simulink model "PDUSTM32"  (R2024b)
settings: Solver=FixedStepDiscrete  StartTime=0.0  StopTime=1  FixedStep=0.001  RelTol=1e-3  EnableMultiTasking=on
libraries: stm32blockslib x24, stm32f4xxblockslib x11, canmsglib x7, simulink x3, stm32h7xxblockslib x1
settings Model: STM32="{\"DigitalPortRead\":{\"ID\":\"PDUSTM32:620\"},\"SPIControllerTransfer\":[{\"ID\":\"PDUSTM32:616\"},{\"ID\":\"PDUSTM32:709\"},{\"ID\":\"PDUSTM32:716\"},{\"ID\":\"PDUSTM32:722\"},{\"ID\":\"PDUSTM32:728\"},{\"ID\":\"PDUSTM32:854\"},{\"ID\":\"PDUSTM32:855\"},{\"ID\":\"PDUSTM32:867\"},{\"ID\":\"PDUSTM32:868\"},{\"ID\":\"PDUSTM32:880\"},{\"ID\":\"PDUSTM32:881\"},{\"ID\":\"PDUSTM32:1012\"},{\"ID\":\"PDUSTM32:1013\"},{\"ID\":\"PDUSTM32:1014\"},{\"ID\":\"PDUSTM32:1015\"},{\"ID\":\"PDUSTM32:1016\"},{\"ID\":\"PDUSTM32:1017\"},{\"ID\":\"PDUSTM32:1018\"},{\"ID\":\"PDUSTM32:1019\"},{\"ID\":\"PDUSTM32:1077\"},{\"ID\":\"PDUSTM32:1078\"},{\"ID\":\"PDUSTM32:1090\"},{\"ID\":\"PDUSTM32:1109\"},{\"ID\":\"PDUSTM32:1110\"}],\"AnalogInputForH7\":{\"ID\":\"PDUSTM32:731\"},\"DigitalPortWrite\":[{\"ID\":\"PDUSTM32:809\"},{\"ID\":\"PDUSTM32:825\"},{\"ID\":\"PDUSTM32:826\"},{\"ID\":\"PDUSTM32:889\"},{\"ID\":\"PDUSTM32:921\"},{\"ID\":\"PDUSTM32:1091\"},{\"ID\":\"PDUSTM32:1092\"},{\"ID\":\"PDUSTM32:1093\"},{\"ID\":\"PDUSTM32:1094\"},{\"ID\":\"PDUSTM32:1095\"}]}"  Creator=will  LastModifiedBy=Will
settings SolverCC: AlgebraicLoopSolver=TrustRegion
settings DataIOCC: ReturnWorkspaceOutputs=off
settings OptimizationCC: DefaultParameterBehavior=Inlined  EnhancedBackFolding=on  PassReuseOutputArgsAs=Individual arguments  ZeroExternalMemoryAtStartup=off  ZeroInternalMemoryAtStartup=off  MaxStackSize=512  OptimizeBlockOrder=speed  DifferentSizesBufferReuse=on  OptimizationCustomize=off  EfficientTunableParamExpr=on
settings DebuggingCC: ParameterTunabilityLossMsg=error  UnconnectedInputMsg=warning  UnconnectedOutputMsg=warning  UnconnectedLineMsg=warning  ArithmeticOperatorsInVariantConditions=warning
settings HardwareCC: ProdBitPerPointer=32  ProdBitPerSizeT=32  ProdBitPerPtrDiffT=32  ProdLargestAtomicInteger=Long  ProdLargestAtomicFloat=Double  ProdWordSize=32  ProdLongLongMode=on  ProdHWDeviceType=ARM Compatible->ARM Cortex-M
settings ModelReferenceCC: EnableRefExpFcnMdlSchedulingChecks=on
settings SFSimCC: MATLABDynamicMemAlloc=off  CustomCodeUndefinedFunction=UseInterfaceOnly
settings RTWCC: Description=Embedded Coder  SystemTargetFile=ert.tlc  HardwareBoard=STM32H7xx Based (Single-core)  TemplateMakefile=ert_default_tmf  CustomHeaderCode="#include \"stm32h7xx_ll_tim.h\""  CustomInitializer=LL_TIM_EnableCounter(TIM2);  Toolchain=GNU Tools for ARM Embedded Processors  GPUComputeCapability=3.5
settings CodeAppCC: ForceParamTrailComments=on  IgnoreCustomStorageClasses=off  OperatorAnnotations=on  SimulinkDataObjDesc=on  SFDataObjDesc=on  InsertBlockDesc=on
settings ERTTargetCC: TargetLangStandard=C99 (ISO)  CodeReplacementLibrary=ARM Cortex-M  ExtModeTransport=3  ExtModeStaticAlloc=on  ExtModeStaticAllocSize=2048  ExtModeMexFile=ext_xcp  ExtModeIntrfLevel=Level2 - Open

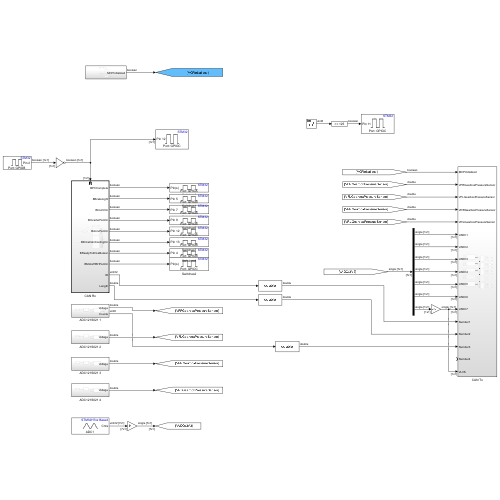
[thumbnail: Simulink's stored preview of the top-level diagram]
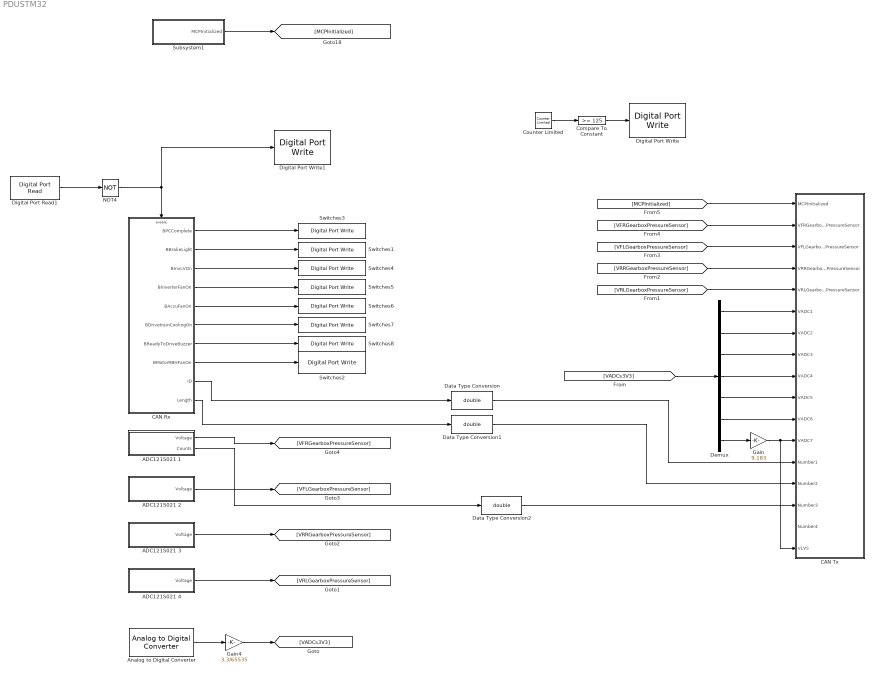
== system PDUSTM32 ==
  ADC121S021 1 : Subsystem
  ADC121S021 2 : Subsystem
  ADC121S021 3 : Subsystem
  ADC121S021 4 : Subsystem
  Analog to Digital Converter : stm32h7xxblockslib/Analog to Digital Converter  ADCModule=ADC1  ConversionGroup=Regular  TriggerMode=Read results only  NumberOfConversions=7  EnableBufferConv=off  BufferLength=1  OutputStatus=off  SampleTime=-1  EnableSimPort=off  hoistedMaskSrc=ECSoC/ECSimCodegen/Analog to Digital Converter
  CAN Rx : Subsystem  TreatAsAtomicUnit=on
  CAN Tx : Subsystem
  Compare To Constant : simulink/Logic and Bit Operations/Compare To Constant  relop=>=  const=125  OutDataTypeStr=boolean
  Counter Limited : simulink/Sources/Counter Limited  uplimit=250  tsamp=-1
  Data Type Conversion : DataTypeConversion  OutDataTypeStr=double  SaturateOnIntegerOverflow=off  RndMeth=Floor
  Data Type Conversion1 : DataTypeConversion  OutDataTypeStr=double  SaturateOnIntegerOverflow=off  RndMeth=Floor
  Data Type Conversion2 : DataTypeConversion  OutDataTypeStr=double  SaturateOnIntegerOverflow=off  RndMeth=Floor
  Demux : Demux  Outputs=7
  Digital Port Read1 : stm32f4xxblockslib/Digital Port Read  PortName=GPIOB  PinNumber=2  ReadOperation=on  IOAsArray=off  SampleTime=-1  EnableSimPort=off  hoistedMaskSrc=ECSoC/ECSimCodegen/Digital Port Read
      settings: LibrarySourceBlock=stm32f2xxblockslib/Digital Port Read
  Digital Port Write : stm32f4xxblockslib/Digital Port Write  PortName=GPIOC  PinNumber=11  ReadOperation=off  IOAsArray=off  EnableSimPort=off  hoistedMaskSrc=ECSoC/ECSimCodegen/Digital Port Write
      settings: LibrarySourceBlock=stm32h7xxblockslib/Digital Port Write
  Digital Port Write1 : stm32f4xxblockslib/Digital Port Write  PortName=GPIOC  PinNumber=12  ReadOperation=off  IOAsArray=off  EnableSimPort=off  hoistedMaskSrc=ECSoC/ECSimCodegen/Digital Port Write
      settings: LibrarySourceBlock=stm32h7xxblockslib/Digital Port Write
  Gain : Gain  Gain=9.183
  Gain4 : Gain  Gain=3.3/65535  OutDataTypeStr=single
  NOT4 : Logic  Operator=NOT  IconShape=distinctive  AllPortsSameDT=off  OutDataTypeStr=boolean
  Subsystem1 : Subsystem
  Switches1 : stm32f4xxblockslib/Digital Port Write  PortName=GPIOB  PinNumber=5  ReadOperation=off  IOAsArray=off  EnableSimPort=off  hoistedMaskSrc=ECSoC/ECSimCodegen/Digital Port Write
      settings: LibrarySourceBlock=stm32h7xxblockslib/Digital Port Write
  Switches2 : stm32f4xxblockslib/Digital Port Write  PortName=GPIOC  PinNumber=[2]  ReadOperation=off  IOAsArray=on  EnableSimPort=off  hoistedMaskSrc=ECSoC/ECSimCodegen/Digital Port Write
      settings: LibrarySourceBlock=stm32h7xxblockslib/Digital Port Write
  Switches3 : stm32f4xxblockslib/Digital Port Write  PortName=GPIOA  PinNumber=[12]  ReadOperation=off  IOAsArray=on  EnableSimPort=off  hoistedMaskSrc=ECSoC/ECSimCodegen/Digital Port Write
      settings: LibrarySourceBlock=stm32h7xxblockslib/Digital Port Write
  Switches4 : stm32f4xxblockslib/Digital Port Write  PortName=GPIOB  PinNumber=7  ReadOperation=off  IOAsArray=off  EnableSimPort=off  hoistedMaskSrc=ECSoC/ECSimCodegen/Digital Port Write
      settings: LibrarySourceBlock=stm32h7xxblockslib/Digital Port Write
  Switches5 : stm32f4xxblockslib/Digital Port Write  PortName=GPIOB  PinNumber=9  ReadOperation=off  IOAsArray=off  EnableSimPort=off  hoistedMaskSrc=ECSoC/ECSimCodegen/Digital Port Write
      settings: LibrarySourceBlock=stm32h7xxblockslib/Digital Port Write
  Switches6 : stm32f4xxblockslib/Digital Port Write  PortName=GPIOB  PinNumber=12  ReadOperation=off  IOAsArray=off  EnableSimPort=off  hoistedMaskSrc=ECSoC/ECSimCodegen/Digital Port Write
      settings: LibrarySourceBlock=stm32h7xxblockslib/Digital Port Write
  Switches7 : stm32f4xxblockslib/Digital Port Write  PortName=GPIOB  PinNumber=13  ReadOperation=off  IOAsArray=off  EnableSimPort=off  hoistedMaskSrc=ECSoC/ECSimCodegen/Digital Port Write
      settings: LibrarySourceBlock=stm32h7xxblockslib/Digital Port Write
  Switches8 : stm32f4xxblockslib/Digital Port Write  PortName=GPIOB  PinNumber=4  ReadOperation=off  IOAsArray=off  EnableSimPort=off  hoistedMaskSrc=ECSoC/ECSimCodegen/Digital Port Write
      settings: LibrarySourceBlock=stm32h7xxblockslib/Digital Port Write
  wires:
  NOT4/1 -> CAN Rx/Enable, Digital Port Write1/1
  Digital Port Read1/1 -> NOT4/1
  Analog to Digital Converter/1 -> Gain4/1
  Gain4/1 -> [VADCs3V3]
  [VADCs3V3] -> Demux/1
  ADC121S021 1/1(Voltage) -> [VFRGearboxPressureSensor]
  ADC121S021 2/1(Voltage) -> [VFLGearboxPressureSensor]
  ADC121S021 3/1(Voltage) -> [VRRGearboxPressureSensor]
  ADC121S021 4/1(Voltage) -> [VRLGearboxPressureSensor]
  [VFRGearboxPressureSensor] -> CAN Tx/2(VFRGearboxPressureSensor)
  [VFLGearboxPressureSensor] -> CAN Tx/3(VFLGearboxPressureSensor)
  [VRRGearboxPressureSensor] -> CAN Tx/4(VRRGearboxPressureSensor)
  CAN Rx/1(BPCComplete) -> Switches3/1
  [MCPInitialized] -> CAN Tx/1(MCPInitialized)
  CAN Rx/2(BBrakeLight) -> Switches1/1
  CAN Rx/8(BMotorRBHFanOn) -> Switches2/1
  Subsystem1/1(MCPInitialized) -> [MCPInitialized]
  Counter Limited/1 -> Compare To Constant/1
  Compare To Constant/1 -> Digital Port Write/1
  Demux/7 -> Gain/1
  Demux/6 -> CAN Tx/11(VADC6)
  Demux/5 -> CAN Tx/10(VADC5)
  Demux/4 -> CAN Tx/9(VADC4)
  Demux/3 -> CAN Tx/8(VADC3)
  Demux/2 -> CAN Tx/7(VADC2)
  Demux/1 -> CAN Tx/6(VADC1)
  Gain/1 -> CAN Tx/12(VADC7), CAN Tx/17(VLVS)
  CAN Rx/9(ID) -> Data Type Conversion/1
  [VRLGearboxPressureSensor] -> CAN Tx/5(VRLGearboxPressureSensor)
  Data Type Conversion/1 -> CAN Tx/13(Number1)
  CAN Rx/10(Length) -> Data Type Conversion1/1
  Data Type Conversion1/1 -> CAN Tx/14(Number2)
  CAN Rx/3(BInvLVOn) -> Switches4/1
  CAN Rx/4(BInverterFanOn) -> Switches5/1
  CAN Rx/5(BAccuFanOn) -> Switches6/1
  CAN Rx/6(BDrivetrainCoolingOn) -> Switches7/1
  CAN Rx/7(BReadyToDriveBuzzer) -> Switches8/1
  ADC121S021 1/2(Counts) -> Data Type Conversion2/1
  Data Type Conversion2/1 -> CAN Tx/15(Number3)

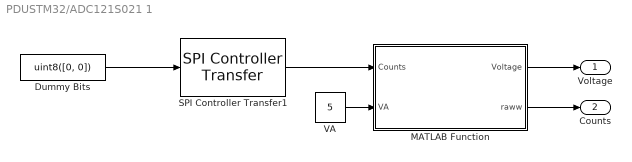
== system PDUSTM32/ADC121S021 1 ==
  Dummy Bits : Constant  Value=uint8([0, 0])
  MATLAB Function : MATLAB Function  TreatAsAtomicUnit=on
  SPI Controller Transfer1 : stm32blockslib/SPI Controller Transfer  Priority=2  SPIModuleSelect=SPI1  ClockPolarity=Low  ClockPhase=1 Edge  SPIModule=uint32(0)  Mode=Master  BusSpeed=uint32(1000000)  FirstBitToTransfer=Most significant bit (MSB)  ClockMode=0  BlockFunction=Transfer  EnableRegisterAddress=off  RegisterAddress=0  OutputDataType=uint8  OutputDataLength=1  OutputStatus=off  BlockingMode=on  Timeout=0.01  DataBits=8  UseCustomSSPin=Explicit GPIO calls  ActiveLowSSPin=Active low  Port_Select=GPIOA  Pin=0
      settings: LibrarySourceBlock=stm32h7xxblockslib/SPI Controller Transfer
  VA : Constant  Value=5  OutDataTypeStr=double
  Voltage : Outport  OutDataTypeStr=double
  Counts : Outport  Port=2  OutDataTypeStr=uint8
  wires:
  Dummy Bits/1 -> SPI Controller Transfer1/1
  SPI Controller Transfer1/1 -> MATLAB Function/1(Counts)
  VA/1 -> MATLAB Function/2(VA)
  MATLAB Function/1(Voltage) -> Voltage/1
  MATLAB Function/2(raww) -> Counts/1

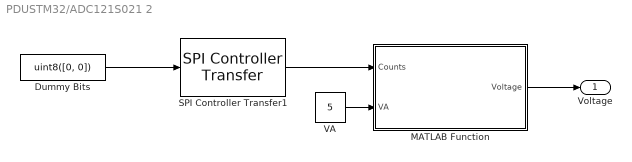
== system PDUSTM32/ADC121S021 2 ==
  Dummy Bits : Constant  Value=uint8([0, 0])
  MATLAB Function : MATLAB Function  TreatAsAtomicUnit=on
  SPI Controller Transfer1 : stm32blockslib/SPI Controller Transfer  Priority=2  SPIModuleSelect=SPI1  ClockPolarity=Low  ClockPhase=1 Edge  SPIModule=uint32(0)  Mode=Master  BusSpeed=uint32(1000000)  FirstBitToTransfer=Most significant bit (MSB)  ClockMode=0  BlockFunction=Transfer  EnableRegisterAddress=off  RegisterAddress=0  OutputDataType=uint8  OutputDataLength=1  OutputStatus=off  BlockingMode=on  Timeout=0.01  DataBits=8  UseCustomSSPin=Explicit GPIO calls  ActiveLowSSPin=Active low  Port_Select=GPIOA  Pin=1
      settings: LibrarySourceBlock=stm32h7xxblockslib/SPI Controller Transfer
  VA : Constant  Value=5
  Voltage : Outport  OutDataTypeStr=double
  wires:
  Dummy Bits/1 -> SPI Controller Transfer1/1
  SPI Controller Transfer1/1 -> MATLAB Function/1(Counts)
  VA/1 -> MATLAB Function/2(VA)
  MATLAB Function/1(Voltage) -> Voltage/1

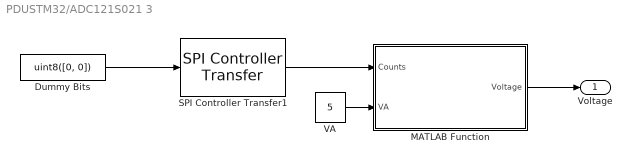
== system PDUSTM32/ADC121S021 3 ==
  Dummy Bits : Constant  Value=uint8([0, 0])
  MATLAB Function : MATLAB Function  TreatAsAtomicUnit=on
  SPI Controller Transfer1 : stm32blockslib/SPI Controller Transfer  Priority=2  SPIModuleSelect=SPI1  ClockPolarity=Low  ClockPhase=1 Edge  SPIModule=uint32(0)  Mode=Master  BusSpeed=uint32(1000000)  FirstBitToTransfer=Most significant bit (MSB)  ClockMode=0  BlockFunction=Transfer  EnableRegisterAddress=off  RegisterAddress=0  OutputDataType=uint8  OutputDataLength=1  OutputStatus=off  BlockingMode=on  Timeout=0.01  DataBits=8  UseCustomSSPin=Explicit GPIO calls  ActiveLowSSPin=Active low  Port_Select=GPIOA  Pin=2
      settings: LibrarySourceBlock=stm32h7xxblockslib/SPI Controller Transfer
  VA : Constant  Value=5
  Voltage : Outport  OutDataTypeStr=double
  wires:
  Dummy Bits/1 -> SPI Controller Transfer1/1
  SPI Controller Transfer1/1 -> MATLAB Function/1(Counts)
  VA/1 -> MATLAB Function/2(VA)
  MATLAB Function/1(Voltage) -> Voltage/1

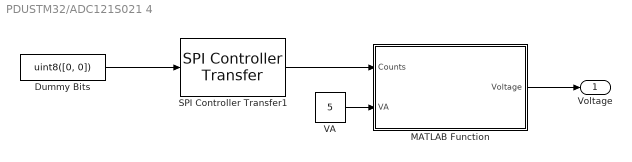
== system PDUSTM32/ADC121S021 4 ==
  Dummy Bits : Constant  Value=uint8([0, 0])
  MATLAB Function : MATLAB Function  TreatAsAtomicUnit=on
  SPI Controller Transfer1 : stm32blockslib/SPI Controller Transfer  Priority=2  SPIModuleSelect=SPI1  ClockPolarity=Low  ClockPhase=1 Edge  SPIModule=uint32(0)  Mode=Master  BusSpeed=uint32(1000000)  FirstBitToTransfer=Most significant bit (MSB)  ClockMode=0  BlockFunction=Transfer  EnableRegisterAddress=off  RegisterAddress=0  OutputDataType=uint8  OutputDataLength=1  OutputStatus=off  BlockingMode=on  Timeout=0.01  DataBits=8  UseCustomSSPin=Explicit GPIO calls  ActiveLowSSPin=Active low  Port_Select=GPIOB  Pin=10
      settings: LibrarySourceBlock=stm32h7xxblockslib/SPI Controller Transfer
  VA : Constant  Value=5
  Voltage : Outport  OutDataTypeStr=double
  wires:
  Dummy Bits/1 -> SPI Controller Transfer1/1
  SPI Controller Transfer1/1 -> MATLAB Function/1(Counts)
  VA/1 -> MATLAB Function/2(VA)
  MATLAB Function/1(Voltage) -> Voltage/1

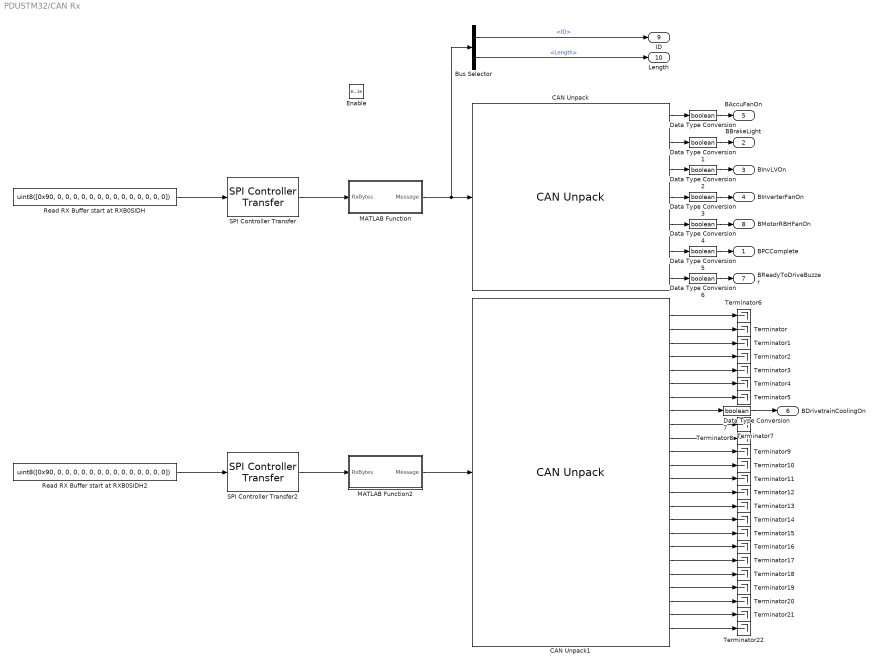
== system PDUSTM32/CAN Rx ==
  Enable : EnablePort
  Bus Selector : BusSelector  OutputSignals=ID,Length
  CAN Unpack : canmsglib/CAN Unpack  CANdbFile=C:\Users\oxbro\Documents\STM32CustomProjects\PDUSTM32\CAN3_28.06.26.dbc  MsgList=VCU_PDMReq  MsgName=VCU_PDMReq  MsgIDType=Standard (11-bit identifier)  MsgIdentifier=1539  MsgLength=7  SignalInfo={'BAccuFanOn','24','1','LE','unsigned','Standard','0','1','0','0','1';'BBrakeLight','0','1','LE','unsigned','Standard','0','1','0','0','1';'BInvLVOn','32','1','LE','unsigned','Standard','0','1','0','0','1';'BInverterFanOn','8','1','LE','unsigned','Standard','0','1','0','0','1';'BMotorRBHFanOn','16','1','LE','unsigned','Standard','0','1','0','0','1';'BPCComplete','40','1','LE','unsigned','Standard','0','1','0','0','1';'BReadyToDriveBuzzer','48','1','LE','unsigned','Standard','0','1','0','0','1'}  IDPort=off  TimestampPort=off  ErrorPort=off  RemotePort=off  LengthPort=off  StatusPort=off  ApplyMinMax=off
      settings: LibrarySourceBlock=stmutilitieslib/CAN Unpack  DataFormat=CANdb specified signals
  CAN Unpack1 : canmsglib/CAN Unpack  CANdbFile=C:\Users\will\Desktop\STM32Projects\PDUSTM32\CAN3_28.06.26.dbc  MsgList=VCU_1s_Frame4  MsgName=VCU_1s_Frame4  MsgIDType=Standard (11-bit identifier)  MsgIdentifier=419  MsgLength=6  SignalInfo={'BBMSP0A0COut','32','1','LE','unsigned','Standard','0','1','0','0','1';'BBMSP0A0EOut','33','1','LE','unsigned','Standard','0','1','0','0','1';'BBMSP0A10Out','34','1','LE','unsigned','Standard','0','1','0','0','1';'BBMSP0A80Out','35','1','LE','unsigned','Standard','0','1','0','0','1';'BBMSP0AC0Out','36','1','LE','unsigned','Standard','0','1','0','0','1';'BBMSP0AFAOut','37','1','LE','unsigned','Standard','0','1','0','0','1';'BBalancingOnOut','31','1','LE','unsigned','Standard','0','1','0','0','1';'BDrivetrainCoolingOn','1','1','LE','unsigned','Standard','0','1','0','0','1';'BDrivetrainCoolingOnEM','5','1','LE','unsigned','Standard','0','1','0','0','1';'BDrivetrainCoolingOnOW','6','2','LE','unsigned','Standard','0','1','-1','-1','2';'BEMSOn','13','1','LE','unsigned','Standard','0','1','0','0','1';'BEMSOnEM','14','1','LE','unsigned','Standard','0','1','0','0','1';'BEMSOnOW','15','2','LE','unsigned','Standard','0','1','-1','-1','2';'BSpinningModeOn','17','1','LE','unsigned','Standard','0','1','0','0','1';'BSpinningModeOnEM','18','1','LE','unsigned','Standard','0','1','0','0','1';'BSpinningModeOnOW','19','2','LE','unsigned','Standard','0','1','-1','-1','2';'BTCOn','9','1','LE','unsigned','Standard','0','1','0','0','1';'BTCOnEM','10','1','LE','unsigned','Standard','0','1','0','0','1';'BTCOnOW','11','2','LE','unsigned','Standard','0','1','-1','-1','2';'BTVOnEM','0','1','LE','unsigned','Standard','0','1','0','0','1';'BTVOnOW','2','2','LE','unsigned','Standard','0','1','-1','-1','2';'NEventMode','44','4','LE','unsigned','Standard','0','1','0','0','15';'NLap','38','6','LE','unsigned','Standard','0','1','0','0','63';'rSoE','21','10','LE','unsigned','Standard','0','0.1','0','0','102.3'}  IDPort=off  TimestampPort=off  ErrorPort=off  RemotePort=off  LengthPort=off  StatusPort=off  ApplyMinMax=off
      settings: LibrarySourceBlock=stmutilitieslib/CAN Unpack  DataFormat=CANdb specified signals
  Data Type Conversion{,1..7} (8 alike) : DataTypeConversion  OutDataTypeStr=boolean  SaturateOnIntegerOverflow=off  RndMeth=Floor
  MATLAB Function : MATLAB Function  TreatAsAtomicUnit=on
  MATLAB Function2 : MATLAB Function  TreatAsAtomicUnit=on
  Read RX Buffer start at RXB0SIDH : Constant  Value=uint8([0x90, 0, 0, 0, 0, 0, 0, 0, 0, 0, 0, 0, 0, 0, 0])
  Read RX Buffer start at RXB0SIDH2 : Constant  Value=uint8([0x90, 0, 0, 0, 0, 0, 0, 0, 0, 0, 0, 0, 0, 0, 0])
  SPI Controller Transfer : stm32blockslib/SPI Controller Transfer  Priority=1  SPIModuleSelect=SPI1  ClockPolarity=Low  ClockPhase=1 Edge  SPIModule=uint32(0)  Mode=Master  BusSpeed=uint32(1000000)  FirstBitToTransfer=Most significant bit (MSB)  ClockMode=0  BlockFunction=Transfer  EnableRegisterAddress=off  RegisterAddress=0  OutputDataType=uint8  OutputDataLength=1  OutputStatus=off  BlockingMode=on  Timeout=0.01  DataBits=8  UseCustomSSPin=Explicit GPIO calls  ActiveLowSSPin=Active low  Port_Select=GPIOB  Pin=14
      settings: LibrarySourceBlock=stm32h7xxblockslib/SPI Controller Transfer
  SPI Controller Transfer2 : stm32blockslib/SPI Controller Transfer  Priority=1  SPIModuleSelect=SPI1  ClockPolarity=Low  ClockPhase=1 Edge  SPIModule=uint32(0)  Mode=Master  BusSpeed=uint32(1000000)  FirstBitToTransfer=Most significant bit (MSB)  ClockMode=0  BlockFunction=Transfer  EnableRegisterAddress=off  RegisterAddress=0  OutputDataType=uint8  OutputDataLength=1  OutputStatus=off  BlockingMode=on  Timeout=0.01  DataBits=8  UseCustomSSPin=Explicit GPIO calls  ActiveLowSSPin=Active low  Port_Select=GPIOB  Pin=14
      settings: LibrarySourceBlock=stm32h7xxblockslib/SPI Controller Transfer
  Terminator{,1..22} (23 alike) : Terminator
  BPCComplete : Outport  OutDataTypeStr=boolean
  BBrakeLight : Outport  Port=2  OutDataTypeStr=boolean
  BInvLVOn : Outport  Port=3  OutDataTypeStr=boolean
  BInverterFanOn : Outport  Port=4  OutDataTypeStr=boolean
  BAccuFanOn : Outport  Port=5  OutDataTypeStr=boolean
  BDrivetrainCoolingOn : Outport  Port=6  OutDataTypeStr=boolean
  BReadyToDriveBuzzer : Outport  Port=7  OutDataTypeStr=boolean
  BMotorRBHFanOn : Outport  Port=8  OutDataTypeStr=boolean
  ID : Outport  Port=9
  Length : Outport  Port=10
  wires:
  Read RX Buffer start at RXB0SIDH/1 -> SPI Controller Transfer/1
  SPI Controller Transfer/1 -> MATLAB Function/1(RxBytes)
  MATLAB Function/1(Message) -> Bus Selector/1, CAN Unpack/1
  CAN Unpack/1 -> Data Type Conversion/1
  CAN Unpack/2 -> Data Type Conversion1/1
  CAN Unpack1/2 -> Terminator/1
  CAN Unpack1/3 -> Terminator1/1
  CAN Unpack1/4 -> Terminator2/1
  CAN Unpack1/5 -> Terminator3/1
  CAN Unpack1/6 -> Terminator4/1
  CAN Unpack1/7 -> Terminator5/1
  CAN Unpack1/9 -> Terminator7/1
  CAN Unpack1/10 -> Terminator8/1
  CAN Unpack1/19 -> Terminator17/1
  CAN Unpack1/18 -> Terminator16/1
  CAN Unpack1/17 -> Terminator15/1
  CAN Unpack1/16 -> Terminator14/1
  CAN Unpack1/15 -> Terminator13/1
  CAN Unpack1/14 -> Terminator12/1
  CAN Unpack1/13 -> Terminator11/1
  CAN Unpack1/12 -> Terminator10/1
  CAN Unpack1/20 -> Terminator18/1
  CAN Unpack1/21 -> Terminator19/1
  CAN Unpack1/22 -> Terminator20/1
  CAN Unpack1/23 -> Terminator21/1
  CAN Unpack1/24 -> Terminator22/1
  CAN Unpack1/11 -> Terminator9/1
  CAN Unpack1/1 -> Terminator6/1
  Data Type Conversion/1 -> BAccuFanOn/1
  Data Type Conversion1/1 -> BBrakeLight/1
  Data Type Conversion2/1 -> BInvLVOn/1
  Data Type Conversion3/1 -> BInverterFanOn/1
  Data Type Conversion4/1 -> BMotorRBHFanOn/1
  Data Type Conversion6/1 -> BReadyToDriveBuzzer/1
  Data Type Conversion7/1 -> BDrivetrainCoolingOn/1
  Data Type Conversion5/1 -> BPCComplete/1
  CAN Unpack1/8 -> Data Type Conversion7/1
  CAN Unpack/7 -> Data Type Conversion6/1
  Bus Selector/1 -> ID/1  "<ID>"
  Bus Selector/2 -> Length/1  "<Length>"
  Read RX Buffer start at RXB0SIDH2/1 -> SPI Controller Transfer2/1
  SPI Controller Transfer2/1 -> MATLAB Function2/1(RxBytes)
  MATLAB Function2/1(Message) -> CAN Unpack1/1
  CAN Unpack/3 -> Data Type Conversion2/1
  CAN Unpack/4 -> Data Type Conversion3/1
  CAN Unpack/5 -> Data Type Conversion4/1
  CAN Unpack/6 -> Data Type Conversion5/1

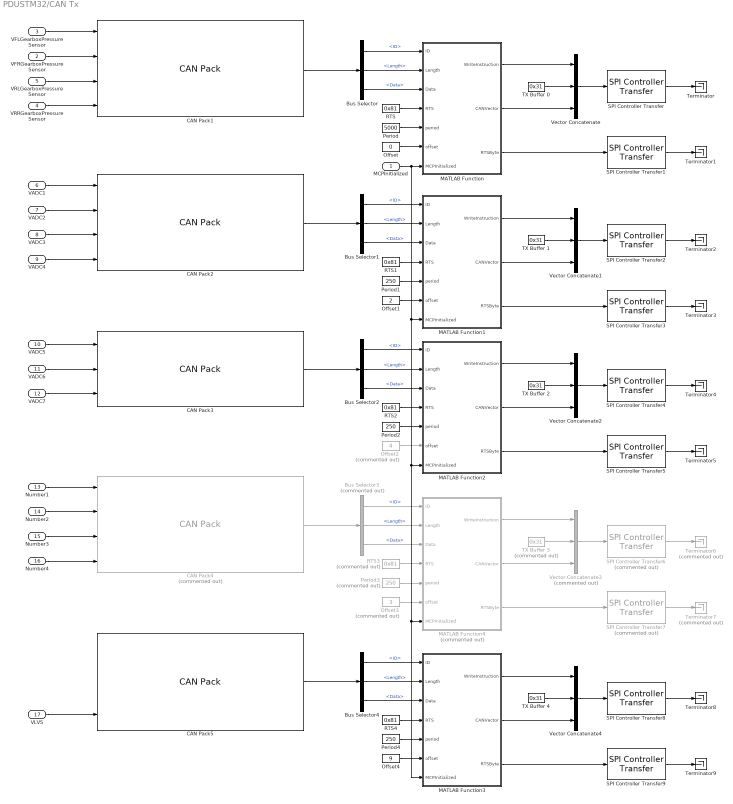
== system PDUSTM32/CAN Tx ==
  MCPInitialized : Inport
  VFRGearboxPressureSensor : Inport  Port=2
  VFLGearboxPressureSensor : Inport  Port=3
  VRRGearboxPressureSensor : Inport  Port=4
  VRLGearboxPressureSensor : Inport  Port=5
  VADC1 : Inport  Port=6
  VADC2 : Inport  Port=7
  VADC3 : Inport  Port=8
  VADC4 : Inport  Port=9
  VADC5 : Inport  Port=10
  VADC6 : Inport  Port=11
  VADC7 : Inport  Port=12
  Number1 : Inport  Port=13
  Number2 : Inport  Port=14
  Number3 : Inport  Port=15
  Number4 : Inport  Port=16
  VLVS : Inport  Port=17
  Bus Selector{,1..2,4} (4 alike) : BusSelector  OutputSignals=ID,Length,Data
  Bus Selector3 : BusSelector  Commented=on  OutputSignals=ID,Length,Data
  CAN Pack1 : canmsglib/CAN Pack  CANdbFile=C:\Users\oxbro\Documents\STM32CustomProjects\PDUSTM32\ADCTest.dbc  MsgList=GearboxPressures  MsgName=GearboxPressures  MsgIDType=Standard (11-bit identifier)  MsgIdentifier=105  CANIDInput=off  MsgLength=8  Remote=off  ApplyMinMax=off  BusOutput=on  SignalInfo={'VFLGearboxPressureSensor','0','12','LE','unsigned','Standard','0','0.0012211','0','0','5.0004';'VFRGearboxPressureSensor','16','12','LE','unsigned','Standard','0','0.0012211','0','0','5.0004';'VRLGearboxPressureSensor','32','12','LE','unsigned','Standard','0','0.0012211','0','0','5.0004';'VRRGearboxPressureSensor','48','12','LE','unsigned','Standard','0','0.0012211','0','0','5.0004'}
      settings: LibrarySourceBlock=stmutilitieslib/CAN Pack  DataFormat=CANdb specified signals
  CAN Pack2 : canmsglib/CAN Pack  CANdbFile=C:\Users\oxbro\Documents\STM32CustomProjects\PDUSTM32\ADCTest.dbc  MsgList=ADCs1  MsgName=ADCs1  MsgIDType=Standard (11-bit identifier)  MsgIdentifier=5  CANIDInput=off  MsgLength=8  Remote=off  ApplyMinMax=off  BusOutput=on  SignalInfo={'VADC1','0','16','LE','unsigned','Standard','0','5.04e-05','0','0','3.303';'VADC2','16','16','LE','unsigned','Standard','0','5.04e-05','0','0','3.303';'VADC3','32','16','LE','unsigned','Standard','0','5.04e-05','0','0','3.303';'VADC4','48','16','LE','unsigned','Standard','0','5.04e-05','0','0','3.303'}
      settings: LibrarySourceBlock=stmutilitieslib/CAN Pack  DataFormat=CANdb specified signals
  CAN Pack3 : canmsglib/CAN Pack  CANdbFile=C:\Users\oxbro\Documents\STM32CustomProjects\PDUSTM32\ADCTest.dbc  MsgList=ADCs2  MsgName=ADCs2  MsgIDType=Standard (11-bit identifier)  MsgIdentifier=66  CANIDInput=off  MsgLength=6  Remote=off  ApplyMinMax=off  BusOutput=on  SignalInfo={'VADC5','0','16','LE','unsigned','Standard','0','5.04e-05','0','0','3.303';'VADC6','16','16','LE','unsigned','Standard','0','5.04e-05','0','0','3.303';'VLVSystem','32','16','LE','unsigned','Standard','0','0.00046327','0','0','30.3604'}
      settings: LibrarySourceBlock=stmutilitieslib/CAN Pack  DataFormat=CANdb specified signals
  CAN Pack4 : canmsglib/CAN Pack  Commented=on  CANdbFile=C:\Users\oxbro\Documents\STM32CustomProjects\PDUSTM32\ADCTest.dbc  MsgList=Numbers  MsgName=Numbers  MsgIDType=Standard (11-bit identifier)  MsgIdentifier=0  CANIDInput=off  MsgLength=8  Remote=off  ApplyMinMax=off  BusOutput=on  SignalInfo={'Number1','0','16','LE','signed','Standard','0','1','0','-32768','32767';'Number2','16','16','LE','signed','Standard','0','1','0','-32768','32767';'Number3','32','16','LE','signed','Standard','0','1','0','-32768','32767';'Number4','48','16','LE','signed','Standard','0','1','0','-32768','32767'}
      settings: LibrarySourceBlock=stmutilitieslib/CAN Pack  DataFormat=CANdb specified signals
  CAN Pack5 : canmsglib/CAN Pack  CANdbFile=C:\Users\Will\Desktop\OBR\Embedded\PDUSTM32\CAN3_28.06.26.dbc  MsgList=PDM_Data  MsgName=PDM_Data  MsgIDType=Standard (11-bit identifier)  MsgIdentifier=1328  CANIDInput=off  MsgLength=8  Remote=off  ApplyMinMax=off  BusOutput=on  SignalInfo={'ILVS','8','8','LE','unsigned','Standard','0','1','0','0','255';'TPDM','16','8','LE','unsigned','Standard','0','1','0','0','255';'VLVS','0','8','LE','unsigned','Standard','0','0.1216','0','0','31.008'}
      settings: LibrarySourceBlock=stmutilitieslib/CAN Pack  DataFormat=CANdb specified signals
  MATLAB Function : MATLAB Function  TreatAsAtomicUnit=on
  MATLAB Function1 : MATLAB Function  TreatAsAtomicUnit=on
  MATLAB Function2 : MATLAB Function  TreatAsAtomicUnit=on
  MATLAB Function3 : MATLAB Function  TreatAsAtomicUnit=on
  MATLAB Function4 : MATLAB Function  Commented=on  TreatAsAtomicUnit=on
  Offset : Constant  Value=0  OutDataTypeStr=uint16  SampleTime=-1
  Offset1 : Constant  Value=2  OutDataTypeStr=uint16  SampleTime=-1
  Offset2 : Constant  Commented=on  Value=4  OutDataTypeStr=uint16  SampleTime=-1
  Offset3 : Constant  Commented=on  Value=3  OutDataTypeStr=uint16  SampleTime=-1
  Offset4 : Constant  Value=9  OutDataTypeStr=uint16  SampleTime=-1
  Period : Constant  Value=5000  OutDataTypeStr=uint16  SampleTime=-1
  Period1 : Constant  Value=250  OutDataTypeStr=uint16  SampleTime=-1
  Period2 : Constant  Value=250  OutDataTypeStr=uint16  SampleTime=-1
  Period3 : Constant  Commented=on  Value=250  OutDataTypeStr=uint16  SampleTime=-1
  Period4 : Constant  Value=250  OutDataTypeStr=uint16  SampleTime=-1
  RTS{,1..2,4} (4 alike) : Constant  Value=0x81  OutDataTypeStr=uint8  SampleTime=-1
  RTS3 : Constant  Commented=on  Value=0x81  OutDataTypeStr=uint8  SampleTime=-1
  SPI Controller Transfer{,2,4,8} (4 alike) : stm32blockslib/SPI Controller Transfer  Priority=1  SPIModuleSelect=SPI1  ClockPolarity=Low  ClockPhase=1 Edge  SPIModule=uint32(0)  Mode=Master  BusSpeed=uint32(1000000)  FirstBitToTransfer=Most significant bit (MSB)  ClockMode=0  BlockFunction=Transfer  EnableRegisterAddress=off  RegisterAddress=0  OutputDataType=uint8  OutputDataLength=1  OutputStatus=off  BlockingMode=off  Timeout=0.01  DataBits=8  UseCustomSSPin=Explicit GPIO calls  ActiveLowSSPin=Active low  Port_Select=GPIOB  Pin=14
      settings: LibrarySourceBlock=stm32h7xxblockslib/SPI Controller Transfer
  SPI Controller Transfer{1,3,5,9} (4 alike) : stm32blockslib/SPI Controller Transfer  Priority=2  SPIModuleSelect=SPI1  ClockPolarity=Low  ClockPhase=1 Edge  SPIModule=uint32(0)  Mode=Master  BusSpeed=uint32(1000000)  FirstBitToTransfer=Most significant bit (MSB)  ClockMode=0  BlockFunction=Transfer  EnableRegisterAddress=off  RegisterAddress=0  OutputDataType=uint8  OutputDataLength=1  OutputStatus=off  BlockingMode=off  Timeout=0.01  DataBits=8  UseCustomSSPin=Explicit GPIO calls  ActiveLowSSPin=Active low  Port_Select=GPIOB  Pin=14
      settings: LibrarySourceBlock=stm32h7xxblockslib/SPI Controller Transfer
  SPI Controller Transfer6 : stm32blockslib/SPI Controller Transfer  Priority=1  Commented=on  SPIModuleSelect=SPI1  ClockPolarity=Low  ClockPhase=1 Edge  SPIModule=uint32(0)  Mode=Master  BusSpeed=uint32(1000000)  FirstBitToTransfer=Most significant bit (MSB)  ClockMode=0  BlockFunction=Transfer  EnableRegisterAddress=off  RegisterAddress=0  OutputDataType=uint8  OutputDataLength=1  OutputStatus=off  BlockingMode=off  Timeout=0.01  DataBits=8  UseCustomSSPin=Explicit GPIO calls  ActiveLowSSPin=Active low  Port_Select=GPIOB  Pin=14
      settings: LibrarySourceBlock=stm32h7xxblockslib/SPI Controller Transfer
  SPI Controller Transfer7 : stm32blockslib/SPI Controller Transfer  Priority=2  Commented=on  SPIModuleSelect=SPI1  ClockPolarity=Low  ClockPhase=1 Edge  SPIModule=uint32(0)  Mode=Master  BusSpeed=uint32(1000000)  FirstBitToTransfer=Most significant bit (MSB)  ClockMode=0  BlockFunction=Transfer  EnableRegisterAddress=off  RegisterAddress=0  OutputDataType=uint8  OutputDataLength=1  OutputStatus=off  BlockingMode=off  Timeout=0.01  DataBits=8  UseCustomSSPin=Explicit GPIO calls  ActiveLowSSPin=Active low  Port_Select=GPIOB  Pin=14
      settings: LibrarySourceBlock=stm32h7xxblockslib/SPI Controller Transfer
  TX Buffer {0..2,4} (4 alike) : Constant  Value=0x31  OutDataTypeStr=uint8  SampleTime=-1
  TX Buffer 3 : Constant  Commented=on  Value=0x31  OutDataTypeStr=uint8  SampleTime=-1
  Terminator{,1..5,8..9} (8 alike) : Terminator
  Terminator6 : Terminator  Commented=on
  Terminator7 : Terminator  Commented=on
  Vector Concatenate{,1..2,4} (4 alike) : Concatenate  NumInputs=3
  Vector Concatenate3 : Concatenate  Commented=on  NumInputs=3
  wires:
  SPI Controller Transfer/1 -> Terminator/1
  MATLAB Function/1(WriteInstruction) -> Vector Concatenate/1
  RTS/1 -> MATLAB Function/4(RTS)
  MATLAB Function/2(CANVector) -> Vector Concatenate/3
  SPI Controller Transfer1/1 -> Terminator1/1
  Bus Selector/1 -> MATLAB Function/1(ID)  "<ID>"
  Vector Concatenate/1 -> SPI Controller Transfer/1
  TX Buffer 0/1 -> Vector Concatenate/2
  MATLAB Function/3(RTSByte) -> SPI Controller Transfer1/1
  Bus Selector/2 -> MATLAB Function/2(Length)  "<Length>"
  Bus Selector/3 -> MATLAB Function/3(Data)  "<Data>"
  CAN Pack1/1 -> Bus Selector/1
  Period/1 -> MATLAB Function/5(period)
  Offset/1 -> MATLAB Function/6(offset)
  VRLGearboxPressureSensor/1 -> CAN Pack1/3
  VRRGearboxPressureSensor/1 -> CAN Pack1/4
  VFRGearboxPressureSensor/1 -> CAN Pack1/2
  VFLGearboxPressureSensor/1 -> CAN Pack1/1
  SPI Controller Transfer2/1 -> Terminator2/1
  SPI Controller Transfer3/1 -> Terminator3/1
  RTS1/1 -> MATLAB Function1/4(RTS)
  MATLAB Function1/2(CANVector) -> Vector Concatenate1/3
  Bus Selector1/3 -> MATLAB Function1/3(Data)  "<Data>"
  Period1/1 -> MATLAB Function1/5(period)
  Bus Selector1/2 -> MATLAB Function1/2(Length)  "<Length>"
  Offset1/1 -> MATLAB Function1/6(offset)
  CAN Pack2/1 -> Bus Selector1/1
  Bus Selector1/1 -> MATLAB Function1/1(ID)  "<ID>"
  MATLAB Function1/3(RTSByte) -> SPI Controller Transfer3/1
  Vector Concatenate1/1 -> SPI Controller Transfer2/1
  MATLAB Function1/1(WriteInstruction) -> Vector Concatenate1/1
  TX Buffer 1/1 -> Vector Concatenate1/2
  SPI Controller Transfer4/1 -> Terminator4/1
  SPI Controller Transfer5/1 -> Terminator5/1
  RTS2/1 -> MATLAB Function2/4(RTS)
  MATLAB Function2/2(CANVector) -> Vector Concatenate2/3
  Bus Selector2/3 -> MATLAB Function2/3(Data)  "<Data>"
  Period2/1 -> MATLAB Function2/5(period)
  Bus Selector2/2 -> MATLAB Function2/2(Length)  "<Length>"
  Offset2/1 -> MATLAB Function2/6(offset)
  CAN Pack3/1 -> Bus Selector2/1
  Bus Selector2/1 -> MATLAB Function2/1(ID)  "<ID>"
  MATLAB Function2/3(RTSByte) -> SPI Controller Transfer5/1
  Vector Concatenate2/1 -> SPI Controller Transfer4/1
  MATLAB Function2/1(WriteInstruction) -> Vector Concatenate2/1
  TX Buffer 2/1 -> Vector Concatenate2/2
  VADC1/1 -> CAN Pack2/1
  VADC2/1 -> CAN Pack2/2
  VADC3/1 -> CAN Pack2/3
  VADC4/1 -> CAN Pack2/4
  VADC5/1 -> CAN Pack3/1
  VADC6/1 -> CAN Pack3/2
  VADC7/1 -> CAN Pack3/3
  Period3/1 -> MATLAB Function4/5(period)
  Vector Concatenate3/1 -> SPI Controller Transfer6/1
  Offset3/1 -> MATLAB Function4/6(offset)
  Number1/1 -> CAN Pack4/1
  MATLAB Function4/3(RTSByte) -> SPI Controller Transfer7/1
  Number4/1 -> CAN Pack4/4
  MATLAB Function4/2(CANVector) -> Vector Concatenate3/3
  Number3/1 -> CAN Pack4/3
  Bus Selector3/3 -> MATLAB Function4/3(Data)  "<Data>"
  Number2/1 -> CAN Pack4/2
  CAN Pack4/1 -> Bus Selector3/1
  Bus Selector3/1 -> MATLAB Function4/1(ID)  "<ID>"
  MATLAB Function4/1(WriteInstruction) -> Vector Concatenate3/1
  TX Buffer 3/1 -> Vector Concatenate3/2
  SPI Controller Transfer6/1 -> Terminator6/1
  SPI Controller Transfer7/1 -> Terminator7/1
  Bus Selector3/2 -> MATLAB Function4/2(Length)  "<Length>"
  RTS3/1 -> MATLAB Function4/4(RTS)
  Period4/1 -> MATLAB Function3/5(period)
  RTS4/1 -> MATLAB Function3/4(RTS)
  Vector Concatenate4/1 -> SPI Controller Transfer8/1
  Offset4/1 -> MATLAB Function3/6(offset)
  Bus Selector4/2 -> MATLAB Function3/2(Length)  "<Length>"
  Bus Selector4/1 -> MATLAB Function3/1(ID)  "<ID>"
  MATLAB Function3/2(CANVector) -> Vector Concatenate4/3
  SPI Controller Transfer8/1 -> Terminator8/1
  MCPInitialized/1 -> MATLAB Function3/7(MCPInitialized), MATLAB Function4/7(MCPInitialized), MATLAB Function2/7(MCPInitialized), MATLAB Function1/7(MCPInitialized), MATLAB Function/7(MCPInitialized)
  Bus Selector4/3 -> MATLAB Function3/3(Data)  "<Data>"
  MATLAB Function3/1(WriteInstruction) -> Vector Concatenate4/1
  SPI Controller Transfer9/1 -> Terminator9/1
  MATLAB Function3/3(RTSByte) -> SPI Controller Transfer9/1
  TX Buffer 4/1 -> Vector Concatenate4/2
  CAN Pack5/1 -> Bus Selector4/1
  VLVS/1 -> CAN Pack5/3

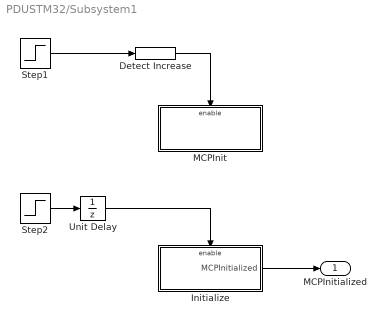
== system PDUSTM32/Subsystem1 ==
  Detect Increase : simulink/Logic and Bit Operations/Detect Increase  vinit=0.0  OutDataTypeStr=boolean
  Initialize : Subsystem  TreatAsAtomicUnit=on
  MCPInit : Subsystem  TreatAsAtomicUnit=on
  Step1 : Step
  Step2 : Step
  Unit Delay : UnitDelay  SampleTime=-1  HasFrameUpgradeWarning=on
  MCPInitialized : Outport
  wires:
  Step1/1 -> Detect Increase/1
  Unit Delay/1 -> Initialize/Enable
  Detect Increase/1 -> MCPInit/Enable
  Step2/1 -> Unit Delay/1
  Initialize/1(MCPInitialized) -> MCPInitialized/1

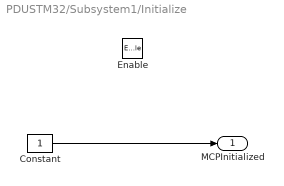
== system PDUSTM32/Subsystem1/Initialize ==
  Enable : EnablePort
  Constant : Constant  OutDataTypeStr=boolean
  MCPInitialized : Outport
  wires:
  Constant/1 -> MCPInitialized/1

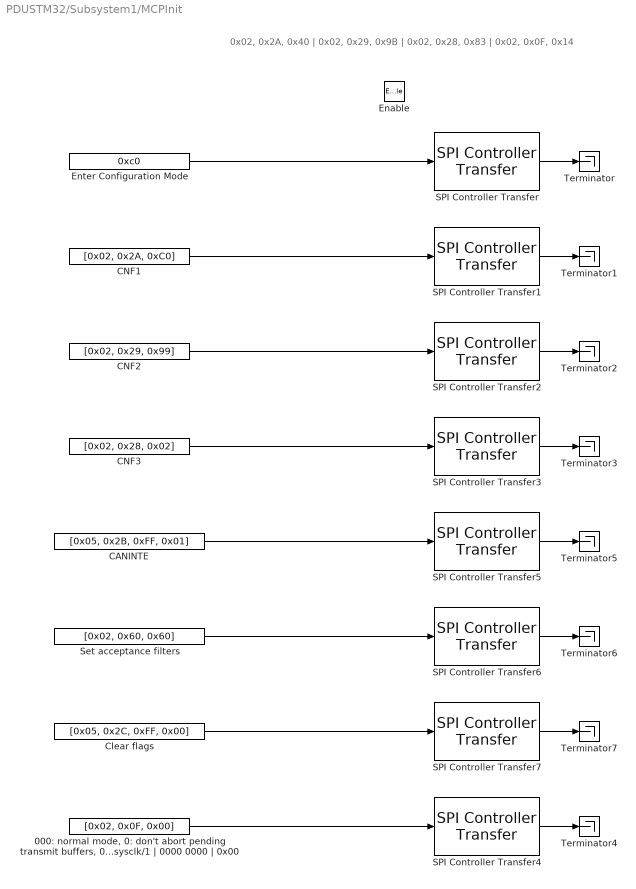
== system PDUSTM32/Subsystem1/MCPInit ==
  note: 0x02, 0x2A, 0x40 | 0x02, 0x29, 0x9B | 0x02, 0x28, 0x83 | 0x02, 0x0F, 0x14
  Enable : EnablePort
  " 000: normal mode, 0: don't abort pending transmit buffers, 0: one-shot disabled, 0: CLKOUT disabled, 00: sysclk/1 | 0000 0000 | 0x00" : Constant  Value=[0x02, 0x0F, 0x00]  OutDataTypeStr=uint8
  CANINTE : Constant  Value=[0x05, 0x2B, 0xFF, 0x01]  OutDataTypeStr=uint8
  CNF1 : Constant  Value=[0x02, 0x2A, 0xC0]  OutDataTypeStr=uint8
  CNF2 : Constant  Value=[0x02, 0x29, 0x99]  OutDataTypeStr=uint8
  CNF3 : Constant  Value=[0x02, 0x28, 0x02]  OutDataTypeStr=uint8
  Clear flags : Constant  Value=[0x05, 0x2C, 0xFF, 0x00]  OutDataTypeStr=uint8
  Enter Configuration Mode : Constant  Value=0xc0  OutDataTypeStr=uint8
  SPI Controller Transfer : stm32blockslib/SPI Controller Transfer  Priority=3  SPIModuleSelect=SPI1  ClockPolarity=Low  ClockPhase=1 Edge  SPIModule=uint32(0)  Mode=Master  BusSpeed=uint32(1000000)  FirstBitToTransfer=Most significant bit (MSB)  ClockMode=0  BlockFunction=Transfer  EnableRegisterAddress=off  RegisterAddress=0  OutputDataType=uint8  OutputDataLength=1  OutputStatus=off  BlockingMode=on  Timeout=0.01  DataBits=8  UseCustomSSPin=Explicit GPIO calls  ActiveLowSSPin=Active low  Port_Select=GPIOB  Pin=14
      settings: LibrarySourceBlock=stm32h7xxblockslib/SPI Controller Transfer
  SPI Controller Transfer1 : stm32blockslib/SPI Controller Transfer  Priority=4  SPIModuleSelect=SPI1  ClockPolarity=Low  ClockPhase=1 Edge  SPIModule=uint32(0)  Mode=Master  BusSpeed=uint32(1000000)  FirstBitToTransfer=Most significant bit (MSB)  ClockMode=0  BlockFunction=Transfer  EnableRegisterAddress=off  RegisterAddress=0  OutputDataType=uint8  OutputDataLength=1  OutputStatus=off  BlockingMode=on  Timeout=0.01  DataBits=8  UseCustomSSPin=Explicit GPIO calls  ActiveLowSSPin=Active low  Port_Select=GPIOB  Pin=14
      settings: LibrarySourceBlock=stm32h7xxblockslib/SPI Controller Transfer
  SPI Controller Transfer2 : stm32blockslib/SPI Controller Transfer  Priority=5  SPIModuleSelect=SPI1  ClockPolarity=Low  ClockPhase=1 Edge  SPIModule=uint32(0)  Mode=Master  BusSpeed=uint32(1000000)  FirstBitToTransfer=Most significant bit (MSB)  ClockMode=0  BlockFunction=Transfer  EnableRegisterAddress=off  RegisterAddress=0  OutputDataType=uint8  OutputDataLength=1  OutputStatus=off  BlockingMode=on  Timeout=0.01  DataBits=8  UseCustomSSPin=Explicit GPIO calls  ActiveLowSSPin=Active low  Port_Select=GPIOB  Pin=14
      settings: LibrarySourceBlock=stm32h7xxblockslib/SPI Controller Transfer
  SPI Controller Transfer3 : stm32blockslib/SPI Controller Transfer  Priority=6  SPIModuleSelect=SPI1  ClockPolarity=Low  ClockPhase=1 Edge  SPIModule=uint32(0)  Mode=Master  BusSpeed=uint32(1000000)  FirstBitToTransfer=Most significant bit (MSB)  ClockMode=0  BlockFunction=Transfer  EnableRegisterAddress=off  RegisterAddress=0  OutputDataType=uint8  OutputDataLength=1  OutputStatus=off  BlockingMode=on  Timeout=0.01  DataBits=8  UseCustomSSPin=Explicit GPIO calls  ActiveLowSSPin=Active low  Port_Select=GPIOB  Pin=14
      settings: LibrarySourceBlock=stm32h7xxblockslib/SPI Controller Transfer
  SPI Controller Transfer4 : stm32blockslib/SPI Controller Transfer  Priority=10  SPIModuleSelect=SPI1  ClockPolarity=Low  ClockPhase=1 Edge  SPIModule=uint32(0)  Mode=Master  BusSpeed=uint32(1000000)  FirstBitToTransfer=Most significant bit (MSB)  ClockMode=0  BlockFunction=Transfer  EnableRegisterAddress=off  RegisterAddress=0  OutputDataType=uint8  OutputDataLength=1  OutputStatus=off  BlockingMode=on  Timeout=0.01  DataBits=8  UseCustomSSPin=Explicit GPIO calls  ActiveLowSSPin=Active low  Port_Select=GPIOB  Pin=14
      settings: LibrarySourceBlock=stm32h7xxblockslib/SPI Controller Transfer
  SPI Controller Transfer5 : stm32blockslib/SPI Controller Transfer  Priority=7  SPIModuleSelect=SPI1  ClockPolarity=Low  ClockPhase=1 Edge  SPIModule=uint32(0)  Mode=Master  BusSpeed=uint32(1000000)  FirstBitToTransfer=Most significant bit (MSB)  ClockMode=0  BlockFunction=Transfer  EnableRegisterAddress=off  RegisterAddress=0  OutputDataType=uint8  OutputDataLength=1  OutputStatus=off  BlockingMode=on  Timeout=0.01  DataBits=8  UseCustomSSPin=Explicit GPIO calls  ActiveLowSSPin=Active low  Port_Select=GPIOB  Pin=14
      settings: LibrarySourceBlock=stm32h7xxblockslib/SPI Controller Transfer
  SPI Controller Transfer6 : stm32blockslib/SPI Controller Transfer  Priority=8  SPIModuleSelect=SPI1  ClockPolarity=Low  ClockPhase=1 Edge  SPIModule=uint32(0)  Mode=Master  BusSpeed=uint32(1000000)  FirstBitToTransfer=Most significant bit (MSB)  ClockMode=0  BlockFunction=Transfer  EnableRegisterAddress=off  RegisterAddress=0  OutputDataType=uint8  OutputDataLength=1  OutputStatus=off  BlockingMode=on  Timeout=0.01  DataBits=8  UseCustomSSPin=Explicit GPIO calls  ActiveLowSSPin=Active low  Port_Select=GPIOB  Pin=14
      settings: LibrarySourceBlock=stm32h7xxblockslib/SPI Controller Transfer
  SPI Controller Transfer7 : stm32blockslib/SPI Controller Transfer  Priority=9  SPIModuleSelect=SPI1  ClockPolarity=Low  ClockPhase=1 Edge  SPIModule=uint32(0)  Mode=Master  BusSpeed=uint32(1000000)  FirstBitToTransfer=Most significant bit (MSB)  ClockMode=0  BlockFunction=Transfer  EnableRegisterAddress=off  RegisterAddress=0  OutputDataType=uint8  OutputDataLength=1  OutputStatus=off  BlockingMode=on  Timeout=0.01  DataBits=8  UseCustomSSPin=Explicit GPIO calls  ActiveLowSSPin=Active low  Port_Select=GPIOB  Pin=14
      settings: LibrarySourceBlock=stm32h7xxblockslib/SPI Controller Transfer
  Set acceptance filters : Constant  Value=[0x02, 0x60, 0x60]  OutDataTypeStr=uint8
  Terminator{,1..7} (8 alike) : Terminator
  wires:
  SPI Controller Transfer7/1 -> Terminator7/1
  CNF3/1 -> SPI Controller Transfer3/1
  SPI Controller Transfer6/1 -> Terminator6/1
  CNF2/1 -> SPI Controller Transfer2/1
  CNF1/1 -> SPI Controller Transfer1/1
  SPI Controller Transfer3/1 -> Terminator3/1
  SPI Controller Transfer1/1 -> Terminator1/1
  Clear flags/1 -> SPI Controller Transfer7/1
  SPI Controller Transfer5/1 -> Terminator5/1
  SPI Controller Transfer2/1 -> Terminator2/1
  " 000: normal mode, 0: don't abort pending transmit buffers, 0: one-shot disabled, 0: CLKOUT disabled, 00: sysclk/1 | 0000 0000 | 0x00"/1 -> SPI Controller Transfer4/1
  SPI Controller Transfer4/1 -> Terminator4/1
  CANINTE/1 -> SPI Controller Transfer5/1
  Set acceptance filters/1 -> SPI Controller Transfer6/1
  Enter Configuration Mode/1 -> SPI Controller Transfer/1
  SPI Controller Transfer/1 -> Terminator/1

== matlab function PDUSTM32/CAN Rx/MATLAB Function2 ==
  data: RxBytes input uint8 size=15; Message output Bus: CAN_MESSAGE_def
function Message = DecodeCANMsg(RxBytes)
%#codegen
% RxBytes is uint8(1x15); bytes 1-2 are don't-care (command echo + one turnaround byte)
SIDH = RxBytes(3);
SIDL = RxBytes(4);
EID8 = RxBytes(5);
EID0 = RxBytes(6);
DLC  = RxBytes(7);

Message.ID       = uint32(bitor(uint32(bitshift(uint32(SIDH), 3)), ...
                        uint32(bitshift(uint32(SIDL), -5))));
Message.Extended = false;
Message.Remote   = false;
Message.Error    = false;
Message.Length   = double(bitand(DLC, uint8(15)));
Message.Data     = RxBytes(8:15);

== matlab function PDUSTM32/CAN Tx/MATLAB Function4 ==
  settings: updateMethod=DISCRETE  sampleTime=.001
  data: WriteInstruction output; ID input uint32; CANVector output uint8; Length input uint8; Data input uint8; RTS input; RTSByte output; period input; offset input; MCPInitialized input
function [WriteInstruction, CANVector, RTSByte] = ConvertToVector(ID, Length, Data, RTS, period, offset, MCPInitialized)
%#codegen
persistent count;
if isempty(count)
    count = uint16(0);
end

if MCPInitialized
    if count == uint16(offset)
        id_u16 = uint16(ID);
        CANVector = zeros(1,13,'uint8');
        CANVector(1) = uint8(bitshift(id_u16, -3));
        CANVector(2) = uint8(bitshift(bitand(id_u16, uint16(7)), 5));
        CANVector(3) = uint8(0);
        CANVector(4) = uint8(0);
        CANVector(5) = bitand(uint8(Length), uint8(15));
        for i = 1:8
            CANVector(5+i) = uint8(Data(i));
        end
        RTSByte = uint8(RTS);
        WriteInstruction = uint8(0x02);
    else
        CANVector = zeros(1,13,'uint8');
        RTSByte = uint8(0x03);
        WriteInstruction = uint8(0x03);
    end

    count = count + uint16(1);
    if count >= uint16(period)
        count = uint16(0);
    end
else
    CANVector = zeros(1,13,'uint8');
    RTSByte = uint8(0x03);
    WriteInstruction = uint8(0x03);
    % don't increment count while MCP not ready
end

== matlab function PDUSTM32/CAN Tx/MATLAB Function ==
  settings: updateMethod=DISCRETE  sampleTime=.001
  data: WriteInstruction output; ID input uint32; CANVector output uint8; Length input uint8; Data input uint8; RTS input; RTSByte output; period input; offset input; MCPInitialized input
function [WriteInstruction, CANVector, RTSByte] = ConvertToVector(ID, Length, Data, RTS, period, offset, MCPInitialized)
%#codegen
persistent count;
if isempty(count)
    count = uint16(0);
end

if MCPInitialized
    if count == uint16(offset)
        id_u16 = uint16(ID);
        CANVector = zeros(1,13,'uint8');
        CANVector(1) = uint8(bitshift(id_u16, -3));
        CANVector(2) = uint8(bitshift(bitand(id_u16, uint16(7)), 5));
        CANVector(3) = uint8(0);
        CANVector(4) = uint8(0);
        CANVector(5) = bitand(uint8(Length), uint8(15));
        for i = 1:8
            CANVector(5+i) = uint8(Data(i));
        end
        RTSByte = uint8(RTS);
        WriteInstruction = uint8(0x02);
    else
        CANVector = zeros(1,13,'uint8');
        RTSByte = uint8(0x03);
        WriteInstruction = uint8(0x03);
    end

    count = count + uint16(1);
    if count >= uint16(period)
        count = uint16(0);
    end
else
    CANVector = zeros(1,13,'uint8');
    RTSByte = uint8(0x03);
    WriteInstruction = uint8(0x03);
    % don't increment count while MCP not ready
end

== matlab function PDUSTM32/ADC121S021 1/MATLAB Function ==
  data: Counts input uint8; Voltage output; VA input double; raww output
function [Voltage, raww]= ConvertToVoltage(Counts, VA)
    raw = uint16(Counts(1)) * 256 + uint16(Counts(2));
    counts = double(bitshift(raw, -1) & uint16(4095));
    Voltage = double(counts * (VA / 4095.0));
    raww = Counts(1);
end

== matlab function PDUSTM32/CAN Rx/MATLAB Function ==
  data: RxBytes input uint8 size=15; Message output Bus: CAN_MESSAGE_def
function Message = DecodeCANMsg(RxBytes)
%#codegen
% RxBytes is uint8(1x15); bytes 1-2 are don't-care (command echo + one turnaround byte)
SIDH = RxBytes(3);
SIDL = RxBytes(4);
EID8 = RxBytes(5);
EID0 = RxBytes(6);
DLC  = RxBytes(7);

Message.ID       = uint32(bitor(uint32(bitshift(uint32(SIDH), 3)), ...
                        uint32(bitshift(uint32(SIDL), -5))));
Message.Extended = false;
Message.Remote   = false;
Message.Error    = false;
Message.Length   = double(bitand(DLC, uint8(15)));
Message.Data     = RxBytes(8:15);

== matlab function PDUSTM32/CAN Tx/MATLAB Function3 ==
  settings: updateMethod=DISCRETE  sampleTime=.001
  data: WriteInstruction output; ID input uint32; CANVector output uint8; Length input uint8; Data input uint8; RTS input; RTSByte output; period input; offset input; MCPInitialized input
function [WriteInstruction, CANVector, RTSByte] = ConvertToVector(ID, Length, Data, RTS, period, offset, MCPInitialized)
%#codegen
persistent count;
if isempty(count)
    count = uint16(0);
end

if MCPInitialized
    if count == uint16(offset)
        id_u16 = uint16(ID);
        CANVector = zeros(1,13,'uint8');
        CANVector(1) = uint8(bitshift(id_u16, -3));
        CANVector(2) = uint8(bitshift(bitand(id_u16, uint16(7)), 5));
        CANVector(3) = uint8(0);
        CANVector(4) = uint8(0);
        CANVector(5) = bitand(uint8(Length), uint8(15));
        for i = 1:8
            CANVector(5+i) = uint8(Data(i));
        end
        RTSByte = uint8(RTS);
        WriteInstruction = uint8(0x02);
    else
        CANVector = zeros(1,13,'uint8');
        RTSByte = uint8(0x03);
        WriteInstruction = uint8(0x03);
    end

    count = count + uint16(1);
    if count >= uint16(period)
        count = uint16(0);
    end
else
    CANVector = zeros(1,13,'uint8');
    RTSByte = uint8(0x03);
    WriteInstruction = uint8(0x03);
    % don't increment count while MCP not ready
end

== matlab function PDUSTM32/ADC121S021 2/MATLAB Function ==
  data: Counts input uint8; Voltage output double; VA input double
function Voltage = ConvertToVoltage(Counts, VA)
    raw = uint16(Counts(1)) * 256 + uint16(Counts(2));
    counts = double(bitshift(raw, -1) & uint16(4095));
    Voltage = double(counts * (VA / 4095.0));
end

== matlab function PDUSTM32/ADC121S021 3/MATLAB Function ==
  data: Counts input uint8; Voltage output double; VA input double
function Voltage = ConvertToVoltage(Counts, VA)
    raw = uint16(Counts(1)) * 256 + uint16(Counts(2));
    counts = double(bitshift(raw, -1) & uint16(4095));
    Voltage = double(counts * (VA / 4095.0));
end

== matlab function PDUSTM32/ADC121S021 4/MATLAB Function ==
  data: Counts input uint8; Voltage output double; VA input double
function Voltage = ConvertToVoltage(Counts, VA)
    raw = uint16(Counts(1)) * 256 + uint16(Counts(2));
    counts = double(bitshift(raw, -1) & uint16(4095));
    Voltage = double(counts * (VA / 4095.0));
end

== matlab function PDUSTM32/CAN Tx/MATLAB Function1 ==
  settings: updateMethod=DISCRETE  sampleTime=.001
  data: WriteInstruction output; ID input uint32; CANVector output uint8; Length input uint8; Data input uint8; RTS input; RTSByte output; period input; offset input; MCPInitialized input
function [WriteInstruction, CANVector, RTSByte] = ConvertToVector(ID, Length, Data, RTS, period, offset, MCPInitialized)
%#codegen
persistent count;
if isempty(count)
    count = uint16(0);
end

if MCPInitialized
    if count == uint16(offset)
        id_u16 = uint16(ID);
        CANVector = zeros(1,13,'uint8');
        CANVector(1) = uint8(bitshift(id_u16, -3));
        CANVector(2) = uint8(bitshift(bitand(id_u16, uint16(7)), 5));
        CANVector(3) = uint8(0);
        CANVector(4) = uint8(0);
        CANVector(5) = bitand(uint8(Length), uint8(15));
        for i = 1:8
            CANVector(5+i) = uint8(Data(i));
        end
        RTSByte = uint8(RTS);
        WriteInstruction = uint8(0x02);
    else
        CANVector = zeros(1,13,'uint8');
        RTSByte = uint8(0x03);
        WriteInstruction = uint8(0x03);
    end

    count = count + uint16(1);
    if count >= uint16(period)
        count = uint16(0);
    end
else
    CANVector = zeros(1,13,'uint8');
    RTSByte = uint8(0x03);
    WriteInstruction = uint8(0x03);
    % don't increment count while MCP not ready
end

== matlab function PDUSTM32/CAN Tx/MATLAB Function2 ==
  settings: updateMethod=DISCRETE  sampleTime=.001
  data: WriteInstruction output; ID input uint32; CANVector output uint8; Length input uint8; Data input uint8; RTS input; RTSByte output; period input; offset input; MCPInitialized input
function [WriteInstruction, CANVector, RTSByte] = ConvertToVector(ID, Length, Data, RTS, period, offset, MCPInitialized)
%#codegen
persistent count;
if isempty(count)
    count = uint16(0);
end

if MCPInitialized
    if count == uint16(offset)
        id_u16 = uint16(ID);
        CANVector = zeros(1,13,'uint8');
        CANVector(1) = uint8(bitshift(id_u16, -3));
        CANVector(2) = uint8(bitshift(bitand(id_u16, uint16(7)), 5));
        CANVector(3) = uint8(0);
        CANVector(4) = uint8(0);
        CANVector(5) = bitand(uint8(Length), uint8(15));
        for i = 1:8
            CANVector(5+i) = uint8(Data(i));
        end
        RTSByte = uint8(RTS);
        WriteInstruction = uint8(0x02);
    else
        CANVector = zeros(1,13,'uint8');
        RTSByte = uint8(0x03);
        WriteInstruction = uint8(0x03);
    end

    count = count + uint16(1);
    if count >= uint16(period)
        count = uint16(0);
    end
else
    CANVector = zeros(1,13,'uint8');
    RTSByte = uint8(0x03);
    WriteInstruction = uint8(0x03);
    % don't increment count while MCP not ready
end
